simulink model "LR_3_var15 (1)"  (R2020b)
settings: Solver=VariableStepAuto  StartTime=0.0  StopTime=600  RelTol=1e-3
undefined symbols (not defined in the file or in its folder): DiscIntNeverNeededParam, u1
libraries: simulink x2
settings Model: Creator=SIA  LastModifiedBy=SIA

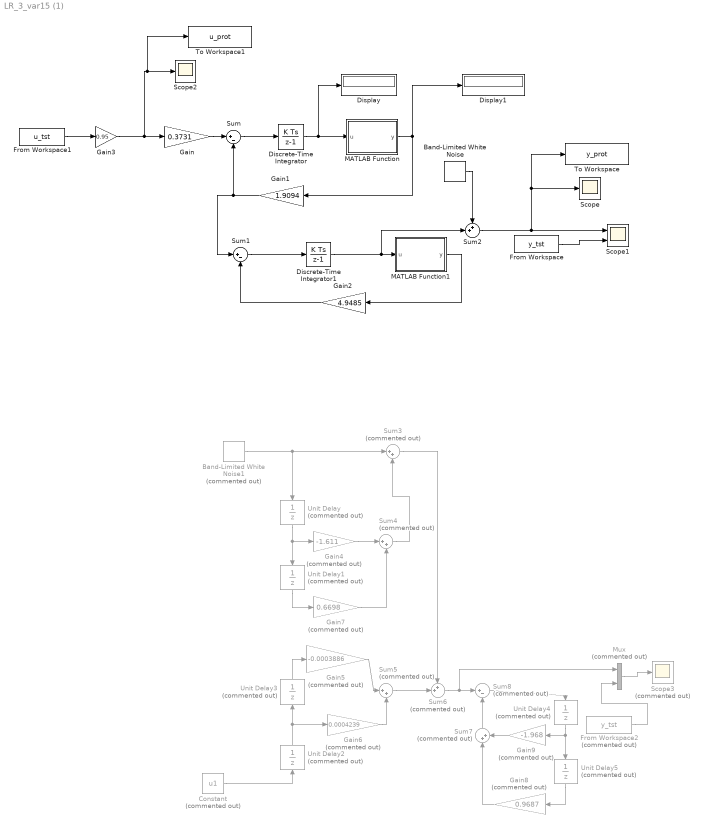
== system LR_3_var15 (1) ==
  Band-Limited White Noise : simulink/Sources/Band-Limited White Noise  Cov=[1e-5]  Ts=0.1  seed=[23341]
  Band-Limited White Noise1 : simulink/Sources/Band-Limited White Noise  Commented=on  Cov=[1e-5]  Ts=0.1  seed=[23341]
  Constant : Constant  Commented=on  Value=u1
  Discrete-Time Integrator : DiscreteIntegrator  gainval=0.234  SampleTime=-1  ICPrevOutput=DiscIntNeverNeededParam  ICPrevScaledInput=DiscIntNeverNeededParam
  Discrete-Time Integrator1 : DiscreteIntegrator  gainval=0.0856  SampleTime=-1  ICPrevOutput=DiscIntNeverNeededParam  ICPrevScaledInput=DiscIntNeverNeededParam
  Display : Display
  Display1 : Display
  From Workspace : FromWorkspace  VariableName=y_tst
  From Workspace1 : FromWorkspace  VariableName=u_tst
  From Workspace2 : FromWorkspace  Commented=on  VariableName=y_tst  SampleTime=-1
  Gain : Gain  Gain=0.3731
  Gain1 : Gain  Gain=1.9094
  Gain2 : Gain  Gain=4.9485
  Gain3 : Gain  Gain=0.95
  Gain4 : Gain  Commented=on  Gain=-1.611
  Gain5 : Gain  Commented=on  Gain=-0.0003886
  Gain6 : Gain  Commented=on  Gain=0.0004239
  Gain7 : Gain  Commented=on  Gain=0.6698
  Gain8 : Gain  Commented=on  Gain=0.9687
  Gain9 : Gain  Commented=on  Gain=-1.968
  MATLAB Function : MATLAB Function  TreatAsAtomicUnit=on
  MATLAB Function1 : MATLAB Function  TreatAsAtomicUnit=on
  Mux : Mux  Commented=on  Inputs=2
  Scope : Scope
  Scope1 : Scope  NumInputPorts=2
  Scope2 : Scope
  Scope3 : Scope  Commented=on
  Sum : Sum  Inputs=|+-
  Sum1 : Sum  Inputs=|+-
  Sum2 : Sum  Inputs=++|
  Sum{3..5,7} (4 alike) : Sum  Commented=on  Inputs=|++
  Sum6 : Sum  Commented=on  Inputs=++|
  Sum8 : Sum  Commented=on  Inputs=|+-
  To Workspace : ToWorkspace  VariableName=y_prot  SaveFormat=Timeseries  SampleTime=0.2
  To Workspace1 : ToWorkspace  VariableName=u_prot  SaveFormat=Timeseries  SampleTime=0.2
  Unit Delay{,1..5} (6 alike) : UnitDelay  Commented=on  SampleTime=-1  HasFrameUpgradeWarning=on
  wires:
  Gain/1 -> Sum/1
  Sum/1 -> Discrete-Time Integrator/1
  Discrete-Time Integrator/1 -> Display/1, MATLAB Function/1(u)
  MATLAB Function/1(y) -> Display1/1, Gain1/1
  Gain1/1 -> Sum/2, Sum1/1
  Gain2/1 -> Sum1/2
  Sum1/1 -> Discrete-Time Integrator1/1
  Band-Limited White Noise/1 -> Sum2/1
  Discrete-Time Integrator1/1 -> MATLAB Function1/1(u), Sum2/2
  MATLAB Function1/1(y) -> Gain2/1
  From Workspace/1 -> Scope1/2
  Sum2/1 -> Scope/1, To Workspace/1, Scope1/1
  Unit Delay/1 -> Gain4/1, Unit Delay1/1
  Band-Limited White Noise1/1 -> Sum3/1, Unit Delay/1
  Gain4/1 -> Sum4/1
  Sum4/1 -> Sum3/2
  Unit Delay2/1 -> Gain6/1, Unit Delay3/1
  Constant/1 -> Unit Delay2/1
  Unit Delay3/1 -> Gain5/1
  Unit Delay1/1 -> Gain7/1
  Gain7/1 -> Sum4/2
  Gain6/1 -> Sum5/2
  Gain5/1 -> Sum5/1
  Sum5/1 -> Sum6/2
  Sum3/1 -> Sum6/1
  Unit Delay4/1 -> Unit Delay5/1, Gain9/1
  Sum8/1 -> Unit Delay4/1
  Unit Delay5/1 -> Gain8/1
  Gain9/1 -> Sum7/2
  Gain8/1 -> Sum7/1
  Sum7/1 -> Sum8/2
  Sum6/1 -> Mux/1, Sum8/1
  From Workspace2/1 -> Mux/2
  Mux/1 -> Scope3/1
  From Workspace1/1 -> Gain3/1
  Gain3/1 -> To Workspace1/1, Scope2/1, Gain/1

== matlab function LR_3_var15 (1)/MATLAB Function ==
  data: u input; y output
function y = fcn(u)
x = u(1);
y = sqrt(x);

== matlab function LR_3_var15 (1)/MATLAB Function1 ==
  data: u input; y output
function y = fcn(u)
x = u(1);
y = sqrt(x);
